simulink model "SF009A_DutyCycThermProtn"  (R2013b)
settings: Solver=FixedStepDiscrete  SolverMode=SingleTasking  StartTime=0.0  StopTime=1  FixedStep=0.1  RelTol=1e-3
values from neighbouring files (symbols this model uses):
  AbsltTThermLimCnt = DataDict.NTC    [SF009A_DutyCycThermProtn_DataDict.m]
  ARCHGLBPRM_100MILLISEC_SEC_F32 = DataDict.Constant    [SF009A_DutyCycThermProtn_DataDict.m]
  CTRLRANDCUTFLT_CNT_U08 = DataDict.Constant    [SF009A_DutyCycThermProtn_DataDict.m]
  CTRLRTFLT_CNT_U08 = DataDict.Constant    [SF009A_DutyCycThermProtn_DataDict.m]
  CUTFLT_CNT_U08 = DataDict.Constant    [SF009A_DutyCycThermProtn_DataDict.m]
  DITHERMLIM_MOTNWTMTR_F32 = DataDict.Constant    [SF009A_DutyCycThermProtn_DataDict.m]
  DutyCycExcddCnt = DataDict.NTC    [SF009A_DutyCycThermProtn_DataDict.m]
  DutyCycThermProtnAbsltCtrlTTblX = DataDict.Calibration    [SF009A_DutyCycThermProtn_DataDict.m]
  DutyCycThermProtnAbsltCtrlTTqTblY = DataDict.Calibration    [SF009A_DutyCycThermProtn_DataDict.m]
  DutyCycThermProtnAbsltCuTTblX = DataDict.Calibration    [SF009A_DutyCycThermProtn_DataDict.m]
  DutyCycThermProtnAbsltCuTTqTblY = DataDict.Calibration    [SF009A_DutyCycThermProtn_DataDict.m]
  DutyCycThermProtnAbsltMotVelBreakPt = DataDict.Calibration    [SF009A_DutyCycThermProtn_DataDict.m]
  DutyCycThermProtnAbsltTTqSlewHiLim = DataDict.Calibration    [SF009A_DutyCycThermProtn_DataDict.m]
  DutyCycThermProtnAbsltTTqSlewLoLim = DataDict.Calibration    [SF009A_DutyCycThermProtn_DataDict.m]
  DutyCycThermProtnCtrlT = DataDict.Calibration    [SF009A_DutyCycThermProtn_DataDict.m]
  DutyCycThermProtnCtrlTSeln = DataDict.Calibration    [SF009A_DutyCycThermProtn_DataDict.m]
  DutyCycThermProtnDutyCycFildThd = DataDict.Calibration    [SF009A_DutyCycThermProtn_DataDict.m]
  DutyCycThermProtnIgnOffCtrlEna = DataDict.Calibration    [SF009A_DutyCycThermProtn_DataDict.m]
  DutyCycThermProtnIgnOffMsgWaitTi = DataDict.Calibration    [SF009A_DutyCycThermProtn_DataDict.m]
  DutyCycThermProtnLstTblValNonStall = DataDict.Calibration    [SF009A_DutyCycThermProtn_DataDict.m]
  DutyCycThermProtnLstTblValStall = DataDict.Calibration    [SF009A_DutyCycThermProtn_DataDict.m]
  DutyCycThermProtnMotPrTSeln = DataDict.Calibration    [SF009A_DutyCycThermProtn_DataDict.m]
  DutyCycThermProtnMplr1NonStallTblY = DataDict.Calibration    [SF009A_DutyCycThermProtn_DataDict.m]
  DutyCycThermProtnMplr1StallTblY = DataDict.Calibration    [SF009A_DutyCycThermProtn_DataDict.m]
  DutyCycThermProtnMplr2NonStallTblY = DataDict.Calibration    [SF009A_DutyCycThermProtn_DataDict.m]
  DutyCycThermProtnMplr2StallTblY = DataDict.Calibration    [SF009A_DutyCycThermProtn_DataDict.m]
  DutyCycThermProtnMplr3NonStallTblY = DataDict.Calibration    [SF009A_DutyCycThermProtn_DataDict.m]
  DutyCycThermProtnMplr3StallTblY = DataDict.Calibration    [SF009A_DutyCycThermProtn_DataDict.m]
  DutyCycThermProtnMplr4NonStallTblY = DataDict.Calibration    [SF009A_DutyCycThermProtn_DataDict.m]
  DutyCycThermProtnMplr4StallTblY = DataDict.Calibration    [SF009A_DutyCycThermProtn_DataDict.m]
  DutyCycThermProtnMplr5NonStallTblY = DataDict.Calibration    [SF009A_DutyCycThermProtn_DataDict.m]
  DutyCycThermProtnMplr5StallTblY = DataDict.Calibration    [SF009A_DutyCycThermProtn_DataDict.m]
  DutyCycThermProtnMplr6NonStallTblY = DataDict.Calibration    [SF009A_DutyCycThermProtn_DataDict.m]
  DutyCycThermProtnMplr6StallTblY = DataDict.Calibration    [SF009A_DutyCycThermProtn_DataDict.m]
  DutyCycThermProtnMplrTblX = DataDict.Calibration    [SF009A_DutyCycThermProtn_DataDict.m]
  DutyCycThermProtnMplrTSeln = DataDict.Calibration    [SF009A_DutyCycThermProtn_DataDict.m]
  DutyCycThermProtnSlowFilTSeln = DataDict.Calibration    [SF009A_DutyCycThermProtn_DataDict.m]
  DutyCycThermProtnThermLimScaFac = DataDict.Calibration    [SF009A_DutyCycThermProtn_DataDict.m]
  DutyCycThermProtnThermLoadLimTblX = DataDict.Calibration    [SF009A_DutyCycThermProtn_DataDict.m]
  DutyCycThermProtnThermLoadLimTblY = DataDict.Calibration    [SF009A_DutyCycThermProtn_DataDict.m]
  DutyCycThermProtnTqCmdSlewDwn = DataDict.Calibration    [SF009A_DutyCycThermProtn_DataDict.m]
  DutyCycThermProtnTqCmdSlewUp = DataDict.Calibration    [SF009A_DutyCycThermProtn_DataDict.m]
  FILVALMIN_ULS_F32 = DataDict.Constant    [SF009A_DutyCycThermProtn_DataDict.m]
  IGNTIOFFTHD_CNT_F32 = DataDict.Constant    [SF009A_DutyCycThermProtn_DataDict.m]
  NODEBSTEP_CNT_U16 = DataDict.Constant    [SF009A_DutyCycThermProtn_DataDict.m]
  ONEPERC_ULS_F32 = DataDict.Constant    [SF009A_DutyCycThermProtn_DataDict.m]
  TAU3_SEC_F32 = DataDict.Constant    [SF009A_DutyCycThermProtn_DataDict.m]
  TAU4_SEC_F32 = DataDict.Constant    [SF009A_DutyCycThermProtn_DataDict.m]
  TAU5_SEC_F32 = DataDict.Constant    [SF009A_DutyCycThermProtn_DataDict.m]
  TAU6_SEC_F32 = DataDict.Constant    [SF009A_DutyCycThermProtn_DataDict.m]
  THERMLOADLIMTBLIDX_ULS_U08 = DataDict.Constant    [SF009A_DutyCycThermProtn_DataDict.m]
undefined symbols (not defined in the file or in its folder): NtcSts1, NvmGetErrSts1
libraries: FixdToFloat x13, Fil x12, NxtrLim x12, simulink x11, NxtrMath x8, FloatToFixd x6, NxtrMax x6, NxtrMin x3, NxtrAbslt x2, NxtrNvM x1
(part 1 of 7)
Description:
  | The purpose of the Thermal Duty Cycle Protection is to limit and protect the system from excessive use,
  | based on motor rotational velocity and system temperature.  It also provides protection status information
  | for use by other functions.
settings Model: ModifiedComment=FZG88Y -- Mon Sep 21 16:56:40 2015 -- Version 1.0.0  Creator=Sneha Pegdal (KPIT)  LastModifiedBy=XZ3VZ1
settings Model: ModifiedHistory=|
  | FZG88Y -- Mon Sep 21 16:56:40 2015 -- Version 1.0.0
  | 
  | 
  | FZG88Y -- Mon Sep 21 16:56:00 2015 -- Version 1.0.0
  | 
  | 
  | FZG88Y -- Mon Sep 21 16:52:01 2015 -- Version 1.0.0
  | 
  | 
  | FZG88Y -- Mon Sep 21 16:48:28 2015 -- Version 1.0.0
  | 
  | 
  | FZG88Y -- Mon Sep 21 16:47:37 2015 -- Version 1.0.0
  | 
  | 
  | FZG88Y -- Mon Sep 21 16:41:44 2015 -- Version 1.0.0
  | 
  | 
  | FZG88Y -- Mon Sep 21 16:36:27 2015 -- Version 1.0.0
  | 
  | 
  | FZG88Y -- Mon Sep 21 16:26:16 2015 -- Version 1.0.0
  | 
  | 
  | FZG88Y -- Mon Sep 21 16:06:23 2015 -- Version 1.0.0
  | 
  | 
  | FZG88Y -- Mon Sep 21 15:59:45 2015 -- Version 1.0.0
  | 
  | 
  | FZG88Y -- Mon Sep 21 15:59:36 2015 -- Version 1.0.0
  | 
  | 
  | FZG88Y -- Mon Sep 21 15:57:42 2015 -- Version 1.0.0
  | 
  | 
  | FZG88Y -- Mon Sep 21 15:57:16 2015 -- Version 1.0.0
  | 
  | 
  | FZG88Y -- Mon Sep 21 15:22:48 2015 -- Version 1.0.0
  | 
  | 
  | FZG88Y -- Mon Sep 21 15:21:30 2015 -- Version 1.0.0
  | 
  | 
  | FZG88Y -- Mon Sep 21 15:21:08 2015 -- Version 1.0.0
  | 
  | 
  | FZG88Y -- Mon Sep 21 15:17:40 2015 -- Version 1.0.0
  | 
  | 
  | FZG88Y -- Mon Sep 21 15:16:45 2015 -- Version 1.0.0
settings SolverCC: AutoInsertRateTranBlk=on  InsertRTBMode=Always
settings DataIOCC: LimitDataPoints=off  SaveFormat=Structure  ReturnWorkspaceOutputs=on
settings OptimizationCC: BlockReduction=off  InlineParams=on  ZeroExternalMemoryAtStartup=off  ZeroInternalMemoryAtStartup=off  OptimizeModelRefInitCode=on  LifeSpan=1
settings DebuggingCC: SignalInfNanChecking=error  SignalRangeChecking=warning  UnderspecifiedInitializationDetection=Simplified  SolverPrmCheckMsg=error  InheritedTsInSrcMsg=error  DiscreteInheritContinuousMsg=error  SingleTaskRateTransMsg=error  TasksWithSamePriorityMsg=error  SigSpecEnsureSampleTimeMsg=error  CheckMatrixSingularityMsg=error  ParameterUnderflowMsg=error  ParameterPrecisionLossMsg=error  ParameterTunabilityLossMsg=error  FixptConstUnderflowMsg=warning  FixptConstOverflowMsg=warning  VectorMatrixConversionMsg=error  SignalLabelMismatchMsg=error  UnconnectedInputMsg=error  UnconnectedOutputMsg=error  UnconnectedLineMsg=error  SFcnCompatibilityMsg=error  UniqueDataStoreMsg=warning  BusObjectLabelMismatch=error  RootOutportRequireBusObject=error  AssertControl=DisableAll  ModelReferenceIOMsg=error  ModelReferenceVersionMismatchMessage=warning  ModelReferenceIOMismatchMessage=error  ModelReferenceCSMismatchMessage=warning  ModelReferenceDataLoggingMessage=error  StateNameClashWarn=warning  StrictBusMsg=ErrorOnBusTreatedAsVector  NonBusSignalsTreatedAsBus=error  SFUnexpectedBacktrackingDiag=error  SFInvalidInputDataAccessInChartInitDiag=error  SFNoUnconditionalDefaultTransitionDiag=error  SFTransitionOutsideNaturalParentDiag=error  SFUnconditionalTransitionShadowingDiag=error  SFUndirectedBroadcastEventsDiag=error
settings ModelReferenceCC: ModelReferenceNumInstancesAllowed=Single
settings RTWCC: SystemTargetFile=autosar.tlc  GenCodeOnly=on  TemplateMakefile=ert_default_tmf  Description=AUTOSAR  GenerateReport=on  ProcessScript=autosar_make_rtw_hook  LaunchReport=on
settings CodeAppCC: GenerateComments=off  IgnoreCustomStorageClasses=off  CustomSymbolStrType=$N$R$M  CustomSymbolStrBlkIO=$N$M  SimulinkBlockComments=off
settings STFCustomTargetCC: ParMdlRefBuildCompliant=on  CompOptLevelCompliant=on  IncludeMdlTerminateFcn=off  CombineOutputUpdateFcns=on  SuppressErrorStatus=on  ERTFirstTimeCompliant=on  ERTCustomFileBanners=on  SupportNonFinite=off  SupportComplex=off  SupportContinuousTime=off  SupportNonInlinedSFcns=off  MATLABClassNameForMDSCustomization=Simulink.SoftwareTarget.ERTCustomization  AutosarCompliant=on  GRTInterface=off  SystemTargetFile=autosar.tlc
settings ERTTargetCC: CodeReplacementLibrary=ANSI_C  ConcurrentExecutionCompliant=off  IncludeMdlTerminateFcn=off  SuppressErrorStatus=on  SupportNonFinite=off  SupportComplex=off  ModelStepFunctionPrototypeControlCompliant=off  CPPClassGenCompliant=off  AutosarCompliant=on  InlinedParameterPlacement=NonHierarchical  ERTCustomFileTemplate=example_file_process.tlc  EnableUserReplacementTypes=on

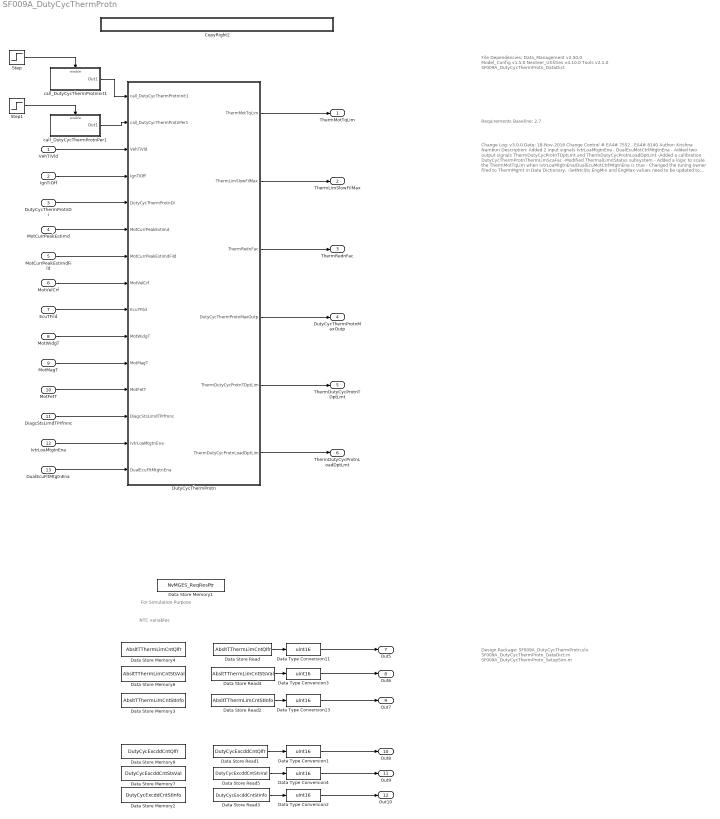
== system SF009A_DutyCycThermProtn ==
  note: For Simulation Purpose
  note: Requirements Baseline: 2.7
  note: File Dependencies:
      |
      | Data_Management v2.50.0
      | Model_Config v1.5.0
      | Nexteer_Utilities v4.10.0
      | Tools v2.1.0
      | SF009A_DutyCycThermProtn_DataDict
  note: Design Package:
      |
      | SF009A_DutyCycThermProtn.slx
      |
      | SF009A_DutyCycThermProtn_DataDict.m
      |
      | SF009A_DutyCycThermProtn_SetupSim.m
  note: NTC variables
  note: Change Log:
      |
      | v3.0.0
      | Date: 18-Nov-2016
      | Change Control # EA4# 7552 , EA4# 8140
      | Author: Krishna Namburi
      | Description:
      | Added 2 input signals IvtrLoaMtgtnEna , DualEcuMotCtrlMtgtnEna
      | - Added two output signals ThermDutyCycProtnTDptLmt and
      | ThermDutyCycProtnLoadDptLmt
      | -Added a calibration DutyCycThermProtnThermLimScaFac
      | -Modified ThermalLimitStatus subsystem
      | - Added a logic to scale the ThermMotTqLim when IvtrLoaMtgtnEna/DualEcuMotCtrlMtgtnEna is true
      | - Changed the tuning owner filed to ThermMgmt in Data Dictionary.
      | -SetNtcSts EngMin and EngMax values need to be updated to match current definition.
      |
      | v2.2.1
      | Date: 21-Sep-2016
      | Change Control # EA4# 7661
      | Author: Krishna Namburi
      | Description:
      | -Added the annotation for look up tables in Multiplier subsystem for
      | Nonstall condition and Stall condition.
      |
      | v2.2.0
      | Date: 05-Aug-2016
      | Change Control #: EA4#6545
      | Author: Fei Yuan
      | Description:
      | - Changed DutyCycThermProtnMplrTblX.Monotony to 'Strictly_Increasing'.
      | - Changed NVM FilStVal.EngInit to blank.
      | - Changed the value of constant CTRLRTFLT_CNT_U08,
      |   CUTFLT_CNT_U08, CTRLRANDCUTFLT_CNT_U08
      | - Added constant NODEBSTEP_CNT_U16
      | - Specified correct bits used in NTCNR_0X0A4 One Pager with new logic to
      |   reach thefull coverage of the MIL test.
      | - Set priority in Init blocks.
      | - Changed NTC names from NTCNR_0X0A3 and NTCNR_0X0A4 to
      |   DutyCycExcddCnt and AbsltTThermLimCnt.
      | - Changed the one-based indexing selectors to zero-based indexing, and
      |   matched the codes.
      | - Changed the DebStep from 0 to NODEBSTEP_CNT_U16 and changed
      |   AbsltTThermLimCnt.NtcTyp to 'None'.
      |
      |
      | v2.1.0
      | Date: 20-Apr-2016
      | Change Control #: EA4#5441
      | Author: Sudeep Shankar
      | Description:
      | - Changed NtcNr1.NTCNR_0X0A4 states:
      | a. 'Prepassed' to 'Passed' and  'Prefailed' to 'Failed' and set debounce step
      | to 0 in the below path:
      | /DutyCycThermProtn/DutyCycThermProtnPer1/TempratureLimiting
      |
      | - Removed ABSLTTTHERMLIMDIAGPASSSTEP_CNT_U16 and
      | ABSLTTTHERMLIMDIAGFAILSTEP_CNT_U16 from DataDictionary as
      | these constants are no longer used.
      |
      | - In Init block, GetErrorStatus block library block is used instead of
      | hardcoded '0' setting to verify NVM validity.
      |
      | - Requirement links to SF009A_132,133,178,179,140 removed as they
      | are no longer applicable
      | - Created requirement links to SF009A_285 and SF009A_138.
      |
      | v2.0.0
      | Date: 04-Apr-2016
      | Change Control #: EA4#5077, EA4#5088
      | Author: Sudeep Shankar
      | Description:
      | EA4#5088:
      | - Removed the calibration DutyCycThermProtnDftIgnOffTi and set
      | the state variables to FILVALMIN_ULS_F32 (0) in the below path:
      | /DutyCycThermProtnPer1/ServiceDefeatFiltSVReinit
      | - Removed DutyCycThermProtnDftIgnOffTi from the DataDictionary.
      |
      | - Constant '0' is changed to defined constant "FILVALMIN_ULS_F32" in
      | the path given below:
      | a.  /DutyCycThermProtnInit1/PowerOnTasks/DefaultIgnOffTime
      | b.  /DutyCycThermProtnPer1/FiltSVReinit/VehTiVldDisabled
      |
      | EA4#5077:
      | -DutyCycThermProtnMaxOutp is added as an output and DataDictionary
      | is updated to include the output signal definition.
      | - Removed display output dDutyCycThermProtnMaxOutp from
      | design and DataDictionary
      |
      | v1.3.0
      | Date: 01-Feb-2015
      | Change Control #: EA4#3601
      | Author: Fei Yuan
      | Description:
      | - Change the logic of NTCs and modify the NTCs definition in the Data
      |   Dictionary.
      | - Add constants CTRLRANDCUTFLT_CNT_U08, CTRLRTFLT_CNT_U08,
      |   CUTFLT_CNT_U08 for NTC.
      |
      | v 1.2.0
      | Date: 09-Dec-2015
      | Chang Control #: EA4#2444
      | Author: Fei Yuan
      | Description
      | - Fixing the the anomaly caused by a floating point exception error by
      |   redesign the logic in PowerOnTasks function and FiltSVReint function.
      | - One constant IGNTIOFFTHD_CNT_F32 is added.
      |
      | v1.1.0
      | Date: 08-Oct-2015
      | Change Control #: EA4#656 (Task EA4#4118)
      | DRW:  Sneha Pegdal/Muragesh Asundi (KPIT)
      | Description:
      | - Data type conversion from float32 to fixed and fixed to float32 before
      |   and after interpolation tables
      | - Debounce logic implemented for NTC 0X0A4
      | - Range limiter added for output ThermRednFac
      | - PIM 'LstTblValRateLimrStVari' is initialized in init function
      |
      | v1.0.0
      | Date: 21-Sept-2015
      | Change Control #: EA4#656 (Task EA4#3734)
      | DRW:  Sneha Pegdal/Muragesh Asundi
      | Description:
      | - Initial Release of EA4 1.0.0 from EA3 V014
  VehTiVld : Inport
  IgnTiOff : Inport  Port=2
  DutyCycThermProtnDi : Inport  Port=3
  MotCurrPeakEstimd : Inport  Port=4
  MotCurrPeakEstimdFild : Inport  Port=5
  MotVelCrf : Inport  Port=6
  EcuTFild : Inport  Port=7
  MotWidgT : Inport  Port=8
  MotMagT : Inport  Port=9
  MotFetT : Inport  Port=10
  DiagcStsLimdTPrfmnc : Inport  Port=11
  IvtrLoaMtgtnEna : Inport  Port=12
  DualEcuFltMtgtnEna : Inport  Port=13
  CopyRight2 : Subsystem  Description=|  mask(Copyright Information){none=on}
      | Copyright info block.                                               
      |                                                                     
      | Place copyright information at the top of every subsystem in design.
      mask prompts: none "No parameters"
      mask help: Place copyright information at the top of every subsystem in design.
      mask Display:
      | NxtrConf = 'Nexteer Confidential';
      | 
      | sys = bdroot; %handle for the current model ("system")
      | first = get_param(sys,'Created');
      | first = first(end-3:end);  %year is last four digits
      | 
      | last = get_param(sys,'LastModifiedDate');
      | if isempty(last)
      |     last = datestr(now,'yyyy');
      | else
      |     last = last(end-3:end);
      | end
      | 
      | if strcmp(first,last)
      |     fprintf('%s -- Copyright %s Nexteer',NxtrConf,first)
      | else
      |     fprintf('%s -- %s%s- %s Nexteer',NxtrConf,char(169),first,last)
      | end
  Data Store Memory1 : DataStoreMemory  DataStoreName=NvMGES_ReqResPtr  OutDataTypeStr=uint8
  Data Store Read : DataStoreRead  DataStoreName=AbsltTThermLimCntQlfr  SampleTime=0.1
  Data Store Read1 : DataStoreRead  DataStoreName=DutyCycExcddCntQlfr  SampleTime=0.1
  Data Store Read2 : DataStoreRead  DataStoreName=AbsltTThermLimCntStInfo  SampleTime=0.1
  Data Store Read3 : DataStoreRead  DataStoreName=DutyCycExcddCntStInfo  SampleTime=0.1
  Data Store Read4 : DataStoreRead  DataStoreName=AbsltTThermLimCntStsVal  SampleTime=0.1
  Data Store Read5 : DataStoreRead  DataStoreName=DutyCycExcddCntStsVal  SampleTime=0.1
  Data Store Memory2 : DataStoreMemory  DataStoreName=DutyCycExcddCntStInfo
  Data Store Memory3 : DataStoreMemory  DataStoreName=AbsltTThermLimCntStInfo
  Data Store Memory4 : DataStoreMemory  DataStoreName=AbsltTThermLimCntQlfr  InitialValue=SigQlfr1.SIGQLFR_NORES  OutDataTypeStr=Enum: SigQlfr1
  Data Store Memory6 : DataStoreMemory  DataStoreName=AbsltTThermLimCntStsVal  InitialValue=NtcSts1.NTCSTS_PASSD  OutDataTypeStr=Enum: NtcSts1
  Data Store Memory7 : DataStoreMemory  DataStoreName=DutyCycExcddCntStsVal  InitialValue=NtcSts1.NTCSTS_PASSD  OutDataTypeStr=Enum: NtcSts1
  Data Store Memory9 : DataStoreMemory  DataStoreName=DutyCycExcddCntQlfr  InitialValue=SigQlfr1.SIGQLFR_NORES  OutDataTypeStr=Enum: SigQlfr1
  Data Type Conversion{1..4,11,13} (6 alike) : DataTypeConversion  OutDataTypeStr=uint16
  DutyCycThermProtn : Subsystem
  Step : Step  Before=1  After=0  SampleTime=0.1
  Step1 : Step  SampleTime=0.1
  call_DutyCycThermProtnInit1 : Subsystem  TreatAsAtomicUnit=on
  call_DutyCycThermProtnPer1 : Subsystem  TreatAsAtomicUnit=on
  ThermMotTqLim : Outport
  ThermLimSlowFilMax : Outport  Port=2
  ThermRednFac : Outport  Port=3
  DutyCycThermProtnMaxOutp : Outport  Port=4
  ThermDutyCycProtnTDptLmt : Outport  Port=5
  ThermDutyCycProtnLoadDptLmt : Outport  Port=6
  Out5 : Outport  Port=7
  Out6 : Outport  Port=8
  Out7 : Outport  Port=9
  Out8 : Outport  Port=10
  Out9 : Outport  Port=11
  Out10 : Outport  Port=12
  wires:
  DutyCycThermProtn/1(ThermMotTqLim) -> ThermMotTqLim/1
  DutyCycThermProtn/2(ThermLimSlowFilMax) -> ThermLimSlowFilMax/1
  DutyCycThermProtn/3(ThermRednFac) -> ThermRednFac/1
  VehTiVld/1 -> DutyCycThermProtn/3(VehTiVld)
  IgnTiOff/1 -> DutyCycThermProtn/4(IgnTiOff)
  DutyCycThermProtnDi/1 -> DutyCycThermProtn/5(DutyCycThermProtnDi)
  MotCurrPeakEstimd/1 -> DutyCycThermProtn/6(MotCurrPeakEstimd)
  MotCurrPeakEstimdFild/1 -> DutyCycThermProtn/7(MotCurrPeakEstimdFild)
  MotVelCrf/1 -> DutyCycThermProtn/8(MotVelCrf)
  EcuTFild/1 -> DutyCycThermProtn/9(EcuTFild)
  MotWidgT/1 -> DutyCycThermProtn/10(MotWidgT)
  MotMagT/1 -> DutyCycThermProtn/11(MotMagT)
  MotFetT/1 -> DutyCycThermProtn/12(MotFetT)
  DiagcStsLimdTPrfmnc/1 -> DutyCycThermProtn/13(DiagcStsLimdTPrfmnc)
  Data Store Read/1 -> Data Type Conversion11/1
  Data Store Read2/1 -> Data Type Conversion13/1
  Data Type Conversion13/1 -> Out7/1
  Data Type Conversion11/1 -> Out5/1
  Data Store Read1/1 -> Data Type Conversion1/1
  Data Store Read3/1 -> Data Type Conversion2/1
  Data Type Conversion2/1 -> Out10/1
  Data Type Conversion1/1 -> Out8/1
  Data Store Read4/1 -> Data Type Conversion3/1
  Data Type Conversion3/1 -> Out6/1
  Data Store Read5/1 -> Data Type Conversion4/1
  Data Type Conversion4/1 -> Out9/1
  DutyCycThermProtn/4(DutyCycThermProtnMaxOutp) -> DutyCycThermProtnMaxOutp/1
  Step/1 -> call_DutyCycThermProtnInit1/Enable
  Step1/1 -> call_DutyCycThermProtnPer1/Enable
  call_DutyCycThermProtnInit1/1(Out1) -> DutyCycThermProtn/1(call_DutyCycThermProtnInit1)
  call_DutyCycThermProtnPer1/1(Out1) -> DutyCycThermProtn/2(call_DutyCycThermProtnPer1)
  DutyCycThermProtn/5(ThermDutyCycProtnTDptLim) -> ThermDutyCycProtnTDptLmt/1
  DutyCycThermProtn/6(ThermDutyCycProtnLoadDptLim) -> ThermDutyCycProtnLoadDptLmt/1
  IvtrLoaMtgtnEna/1 -> DutyCycThermProtn/14(IvtrLoaMtgtnEna)
  DualEcuFltMtgtnEna/1 -> DutyCycThermProtn/15(DualEcuFltMtgtnEna)

== system SF009A_DutyCycThermProtn/CopyRight2 ==

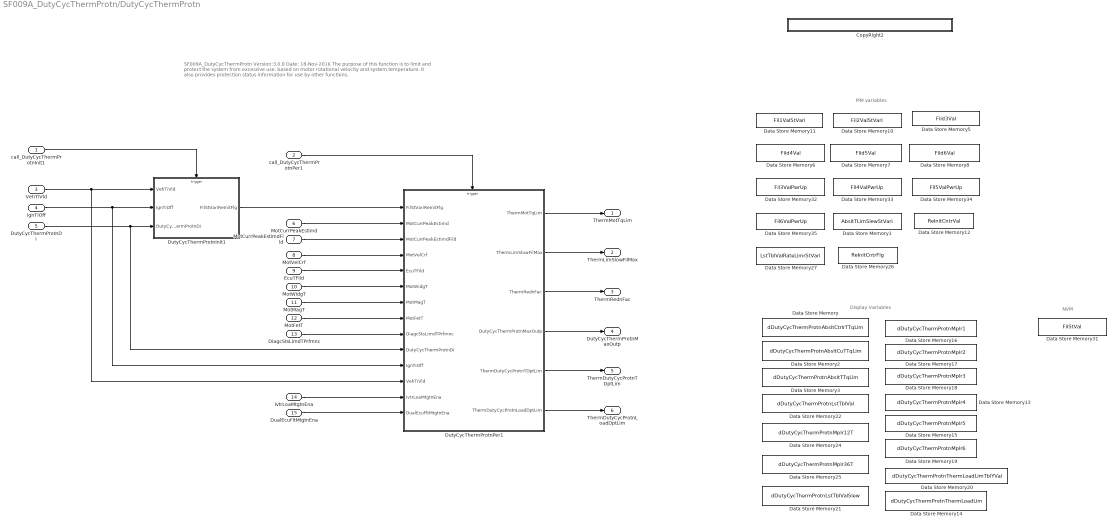
== system SF009A_DutyCycThermProtn/DutyCycThermProtn ==
  note: NVM
  note: Display Variables
  note: PIM variables
  note: SF009A_DutyCycThermProtn      Version:3.0.0                                                 Date:  18-Nov-2016
      | The purpose of this function is to limit and protect the system from excessive use, based on motor rotational velocity and system temperature.
      | It also provides protection status information for use by other functions.
  call_DutyCycThermProtnInit1 : Inport
  call_DutyCycThermProtnPer1 : Inport  Port=2
  VehTiVld : Inport  RequirementInfo={'linktype_rmi_doors' '0000a52a (/E-STEER Core/SubSystem Specifications/Application Functions/SF009A Thermal Duty Cycle Protection)' '#SF009A_39' 'true' 'REQ: SF009A_39' '' } %GIDa_864c1118_778d_4343_bc4d_3cc30f47fe32  Port=3
  IgnTiOff : Inport  RequirementInfo={'linktype_rmi_doors' '0000a52a (/E-STEER Core/SubSystem Specifications/Application Functions/SF009A Thermal Duty Cycle Protection)' '#SF009A_38' 'true' 'REQ: SF009A_38' '' } %GIDa_91c1f96a_b6bf_4566_a475_97c670e9d476  Port=4
  DutyCycThermProtnDi : Inport  RequirementInfo={'linktype_rmi_doors' '0000a52a (/E-STEER Core/SubSystem Specifications/Application Functions/SF009A Thermal Duty Cycle Protection)' '#SF009A_41' 'true' 'REQ: SF009A_41' '' } %GIDa_52de0261_92a3_4db5_85ad_f2cfdd3afac9  Port=5
  MotCurrPeakEstimd : Inport  RequirementInfo={'linktype_rmi_doors' '0000a52a (/E-STEER Core/SubSystem Specifications/Application Functions/SF009A Thermal Duty Cycle Protection)' '#SF009A_9' 'true' 'REQ: SF009A_9' '' } %GIDa_eb01aa28_247f_476b_b7cf_89c03dfe9b33  Port=6
  MotCurrPeakEstimdFild : Inport  RequirementInfo={'linktype_rmi_doors' '0000a52a (/E-STEER Core/SubSystem Specifications/Application Functions/SF009A Thermal Duty Cycle Protection)' '#SF009A_32' 'true' 'REQ: SF009A_32' '' } %GIDa_9a670469_cfaf_4df7_a178_0c897feeb23b  Port=7
  MotVelCrf : Inport  RequirementInfo={'linktype_rmi_doors' '0000a52a (/E-STEER Core/SubSystem Specifications/Application Functions/SF009A Thermal Duty Cycle Protection)' '#SF009A_33' 'true' 'REQ: SF009A_33' '' } %GIDa_17006e69_4cbc_4e82_acf3_d666e95c1429  Port=8
  EcuTFild : Inport  RequirementInfo={'linktype_rmi_doors' '0000a52a (/E-STEER Core/SubSystem Specifications/Application Functions/SF009A Thermal Duty Cycle Protection)' '#SF009A_34' 'true' 'REQ: SF009A_34' '' } %GIDa_c8c2b021_b73b_4c92_8ccd_6e5a076a1f2a  Port=9
  MotWidgT : Inport  RequirementInfo={'linktype_rmi_doors' '0000a52a (/E-STEER Core/SubSystem Specifications/Application Functions/SF009A Thermal Duty Cycle Protection)' '#SF009A_37' 'true' 'REQ: SF009A_37' '' } %GIDa_9410e4a6_6429_4607_8605_4053cc1d35e0  Port=10
  MotMagT : Inport  RequirementInfo={'linktype_rmi_doors' '0000a52a (/E-STEER Core/SubSystem Specifications/Application Functions/SF009A Thermal Duty Cycle Protection)' '#SF009A_36' 'true' 'REQ: SF009A_36' '' } %GIDa_fbe04a47_e117_41dd_aa1c_e1d39b0f3863  Port=11
  MotFetT : Inport  RequirementInfo={'linktype_rmi_doors' '0000a52a (/E-STEER Core/SubSystem Specifications/Application Functions/SF009A Thermal Duty Cycle Protection)' '#SF009A_35' 'true' 'REQ: SF009A_35' '' } %GIDa_71f8b7c1_ac64_4dbe_9e4e_6077f5ec5b92  Port=12
  DiagcStsLimdTPrfmnc : Inport  RequirementInfo={} %GIDa_5be0298f_407d_4486_aa28_f0641ea2ee13  Port=13
  IvtrLoaMtgtnEna : Inport  RequirementInfo={} %GIDa_95a98e68_beb4_4b72_8a6c_64a623d70b4b  Port=14
  DualEcuFltMtgtnEna : Inport  RequirementInfo={} %GIDa_064281bc_c4a7_4daa_abcd_ffd5837e9fb5  Port=15
  CopyRight2 : Subsystem  Description=|  mask(Copyright Information){none=on}
      | Copyright info block.                                               
      |                                                                     
      | Place copyright information at the top of every subsystem in design.
      mask prompts: none "No parameters"
      mask help: Place copyright information at the top of every subsystem in design.
      mask Display:
      | NxtrConf = 'Nexteer Confidential';
      | 
      | sys = bdroot; %handle for the current model ("system")
      | first = get_param(sys,'Created');
      | if(isempty(first))
      |     first = datestr(now,'yyyy');
      | else
      |     first = first(end-3:end);  %year is last four digits
      | end
      | 
      | last = get_param(sys,'LastModifiedDate');
      | if isempty(last)
      |     last = datestr(now,'yyyy');
      | else
      |     last = last(end-3:end);
      | end
      | 
      | if strcmp(first,last)
      |     fprintf('%s -- Copyright %s Nexteer',NxtrConf,first)
      | else
      |     fprintf('%s -- %s%s- %s Nexteer',NxtrConf,char(169),first,last)
      | end
  Data Store Memory : DataStoreMemory  DataStoreName=dDutyCycThermProtnAbsltCtrlrTTqLim  ReadBeforeWriteMsg=warning  WriteAfterWriteMsg=warning  WriteAfterReadMsg=warning  StateMustResolveToSignalObject=on
  Data Store Memory1 : DataStoreMemory  DataStoreName=AbsltTLimSlewStVari  StateMustResolveToSignalObject=on
      settings: AttributesFormatString=Initial Value: %<InitialValue>
  Data Store Memory10 : DataStoreMemory  DataStoreName=Fil2ValStVari  InitialValue=[]  StateMustResolveToSignalObject=on
      settings: AttributesFormatString=Initial Value: %<InitialValue>
  Data Store Memory11 : DataStoreMemory  DataStoreName=Fil1ValStVari  InitialValue=[]  StateMustResolveToSignalObject=on
      settings: AttributesFormatString=Initial Value: %<InitialValue>
  Data Store Memory12 : DataStoreMemory  DataStoreName=ReInitCntrVal  InitialValue=[]  StateMustResolveToSignalObject=on
  Data Store Memory13 : DataStoreMemory  DataStoreName=dDutyCycThermProtnMplr4  ReadBeforeWriteMsg=warning  WriteAfterWriteMsg=warning  WriteAfterReadMsg=warning  StateMustResolveToSignalObject=on
  Data Store Memory14 : DataStoreMemory  DataStoreName=dDutyCycThermProtnThermLoadLim  ReadBeforeWriteMsg=warning  WriteAfterWriteMsg=warning  WriteAfterReadMsg=warning  StateMustResolveToSignalObject=on
  Data Store Memory15 : DataStoreMemory  DataStoreName=dDutyCycThermProtnMplr5  ReadBeforeWriteMsg=warning  WriteAfterWriteMsg=warning  WriteAfterReadMsg=warning  StateMustResolveToSignalObject=on
  Data Store Memory16 : DataStoreMemory  DataStoreName=dDutyCycThermProtnMplr1  ReadBeforeWriteMsg=warning  WriteAfterWriteMsg=warning  WriteAfterReadMsg=warning  StateMustResolveToSignalObject=on
  Data Store Memory17 : DataStoreMemory  DataStoreName=dDutyCycThermProtnMplr2  ReadBeforeWriteMsg=warning  WriteAfterWriteMsg=warning  WriteAfterReadMsg=warning  StateMustResolveToSignalObject=on
  Data Store Memory18 : DataStoreMemory  DataStoreName=dDutyCycThermProtnMplr3  ReadBeforeWriteMsg=warning  WriteAfterWriteMsg=warning  WriteAfterReadMsg=warning  StateMustResolveToSignalObject=on
  Data Store Memory19 : DataStoreMemory  DataStoreName=dDutyCycThermProtnMplr6  ReadBeforeWriteMsg=warning  WriteAfterWriteMsg=warning  WriteAfterReadMsg=warning  StateMustResolveToSignalObject=on
  Data Store Memory2 : DataStoreMemory  DataStoreName=dDutyCycThermProtnAbsltCuTTqLim  ReadBeforeWriteMsg=warning  WriteAfterWriteMsg=warning  WriteAfterReadMsg=warning  StateMustResolveToSignalObject=on
  Data Store Memory20 : DataStoreMemory  DataStoreName=dDutyCycThermProtnThermLoadLimTblYVal  ReadBeforeWriteMsg=warning  WriteAfterWriteMsg=warning  WriteAfterReadMsg=warning  StateMustResolveToSignalObject=on
  Data Store Memory21 : DataStoreMemory  DataStoreName=dDutyCycThermProtnLstTblValSlew  ReadBeforeWriteMsg=warning  WriteAfterWriteMsg=warning  WriteAfterReadMsg=warning  StateMustResolveToSignalObject=on
  Data Store Memory22 : DataStoreMemory  DataStoreName=dDutyCycThermProtnLstTblVal  ReadBeforeWriteMsg=warning  WriteAfterWriteMsg=warning  WriteAfterReadMsg=warning  StateMustResolveToSignalObject=on
  Data Store Memory24 : DataStoreMemory  DataStoreName=dDutyCycThermProtnMplr12T  ReadBeforeWriteMsg=warning  WriteAfterWriteMsg=warning  WriteAfterReadMsg=warning  StateMustResolveToSignalObject=on
  Data Store Memory25 : DataStoreMemory  DataStoreName=dDutyCycThermProtnMplr36T  ReadBeforeWriteMsg=warning  WriteAfterWriteMsg=warning  WriteAfterReadMsg=warning  StateMustResolveToSignalObject=on
  Data Store Memory26 : DataStoreMemory  DataStoreName=ReInitCntrFlg  InitialValue=[]  StateMustResolveToSignalObject=on
  Data Store Memory27 : DataStoreMemory  DataStoreName=LstTblValRateLimrStVari  StateMustResolveToSignalObject=on
      settings: AttributesFormatString=Initial Value: %<InitialValue>
  Data Store Memory3 : DataStoreMemory  DataStoreName=dDutyCycThermProtnAbsltTTqLim  ReadBeforeWriteMsg=warning  WriteAfterWriteMsg=warning  WriteAfterReadMsg=warning  StateMustResolveToSignalObject=on
  Data Store Memory31 : DataStoreMemory  DataStoreName=FilStVal  InitialValue=[]  StateMustResolveToSignalObject=on
      settings: AttributesFormatString=Initial Value: %<InitialValue>
  Data Store Memory32 : DataStoreMemory  DataStoreName=Fil3ValPwrUp  StateMustResolveToSignalObject=on
      settings: AttributesFormatString=Initial Value: %<InitialValue>
  Data Store Memory33 : DataStoreMemory  DataStoreName=Fil4ValPwrUp  StateMustResolveToSignalObject=on
      settings: AttributesFormatString=Initial Value: %<InitialValue>
  Data Store Memory34 : DataStoreMemory  DataStoreName=Fil5ValPwrUp  StateMustResolveToSignalObject=on
      settings: AttributesFormatString=Initial Value: %<InitialValue>
  Data Store Memory35 : DataStoreMemory  DataStoreName=Fil6ValPwrUp  StateMustResolveToSignalObject=on
      settings: AttributesFormatString=Initial Value: %<InitialValue>
  Data Store Memory5 : DataStoreMemory  RequirementInfo={'linktype_rmi_doors' '0000a52a (/E-STEER Core/SubSystem Specifications/Application Functions/SF009A Thermal Duty Cycle Protection)' '#SF009A_285' 'true' 'REQ: SF009A_285' '' } %GIDa_75ef786b_1159_4210_af92_457fb74ea7ff  DataStoreName=Fild3Val  InitialValue=[]  StateMustResolveToSignalObject=on
      settings: AttributesFormatString=Initial Value: %<InitialValue>
  Data Store Memory6 : DataStoreMemory  RequirementInfo={'linktype_rmi_doors' '0000a52a (/E-STEER Core/SubSystem Specifications/Application Functions/SF009A Thermal Duty Cycle Protection)' '#SF009A_285' 'true' 'REQ: SF009A_285' '' } %GIDa_b620ecc7_db63_446e_8f03_37af3e2285f3  DataStoreName=Fild4Val  InitialValue=[]  StateMustResolveToSignalObject=on
      settings: AttributesFormatString=Initial Value: %<InitialValue>
  Data Store Memory7 : DataStoreMemory  RequirementInfo={'linktype_rmi_doors' '0000a52a (/E-STEER Core/SubSystem Specifications/Application Functions/SF009A Thermal Duty Cycle Protection)' '#SF009A_285' 'true' 'REQ: SF009A_285' '' } %GIDa_967c7843_d0f8_4563_990c_866e0e761b03  DataStoreName=Fild5Val  InitialValue=[]  StateMustResolveToSignalObject=on
      settings: AttributesFormatString=Initial Value: %<InitialValue>
  Data Store Memory8 : DataStoreMemory  RequirementInfo={'linktype_rmi_doors' '0000a52a (/E-STEER Core/SubSystem Specifications/Application Functions/SF009A Thermal Duty Cycle Protection)' '#SF009A_285' 'true' 'REQ: SF009A_285' '' } %GIDa_dc28bb5e_67e6_4f32_a254_c55d8b607b43  DataStoreName=Fild6Val  InitialValue=[]  StateMustResolveToSignalObject=on
      settings: AttributesFormatString=Initial Value: %<InitialValue>
  DutyCycThermProtnInit1 : Subsystem  TreatAsAtomicUnit=on
  DutyCycThermProtnPer1 : Subsystem  ClipboardFcn=Priority=%<Priority>  TreatAsAtomicUnit=on
  ThermMotTqLim : Outport  RequirementInfo={'linktype_rmi_doors' '0000a52a (/E-STEER Core/SubSystem Specifications/Application Functions/SF009A Thermal Duty Cycle Protection)' '#SF009A_11' 'true' 'REQ: SF009A_11' '' } %GIDa_b003c252_92e7_4128_b79e_51af7283823f
  ThermLimSlowFilMax : Outport  RequirementInfo={'linktype_rmi_doors' '0000a52a (/E-STEER Core/SubSystem Specifications/Application Functions/SF009A Thermal Duty Cycle Protection)' '#SF009A_44' 'true' 'REQ: SF009A_44' '' } %GIDa_6720560f_cd3f_4a66_9337_c9fda3d2b968  Port=2
  ThermRednFac : Outport  RequirementInfo={'linktype_rmi_doors' '0000a52a (/E-STEER Core/SubSystem Specifications/Application Functions/SF009A Thermal Duty Cycle Protection)' '#SF009A_45' 'true' 'REQ: SF009A_45' '' } %GIDa_bdcba9de_b25d_49eb_95b7_6430acdc662c  Port=3
  DutyCycThermProtnMaxOutp : Outport  RequirementInfo={'linktype_rmi_doors' '0000a52a (/E-STEER Core/SubSystem Specifications/Application Functions/SF009A Thermal Duty Cycle Protection)' '#SF009A_283' 'true' 'REQ: SF009A_283' '' } %GIDa_49eea21d_06a7_40bd_b604_6809298a62bb  Port=4
  ThermDutyCycProtnTDptLim : Outport  RequirementInfo={'linktype_rmi_doors' '0000a52a (/E-STEER Core/SubSystem Specifications/Application Functions/SF009A Thermal Duty Cycle Protection)' '#SF009A_293' 'true' 'REQ: SF009A_293' '' } %GIDa_ce06e884_6156_4583_958e_0184ba4e1972  Port=5
  ThermDutyCycProtnLoadDptLim : Outport  RequirementInfo={'linktype_rmi_doors' '0000a52a (/E-STEER Core/SubSystem Specifications/Application Functions/SF009A Thermal Duty Cycle Protection)' '#SF009A_294' 'true' 'REQ: SF009A_294' '' } %GIDa_34ea47fc_4302_4f6d_8bb6_be5416b6175c  Port=6
  wires:
  call_DutyCycThermProtnPer1/1 -> DutyCycThermProtnPer1/Trigger
  call_DutyCycThermProtnInit1/1 -> DutyCycThermProtnInit1/Trigger
  MotCurrPeakEstimd/1 -> DutyCycThermProtnPer1/2(MotCurrPeakEstimd)
  MotCurrPeakEstimdFild/1 -> DutyCycThermProtnPer1/3(MotCurrPeakEstimdFild)
  MotVelCrf/1 -> DutyCycThermProtnPer1/4(MotVelCrf)
  EcuTFild/1 -> DutyCycThermProtnPer1/5(EcuTFild)
  MotMagT/1 -> DutyCycThermProtnPer1/7(MotMagT)
  DiagcStsLimdTPrfmnc/1 -> DutyCycThermProtnPer1/9(DiagcStsLimdTPrfmnc)
  MotWidgT/1 -> DutyCycThermProtnPer1/6(MotWidgT)
  MotFetT/1 -> DutyCycThermProtnPer1/8(MotFetT)
  VehTiVld/1 -> DutyCycThermProtnInit1/1(VehTiVld), DutyCycThermProtnPer1/12(VehTiVld)
  DutyCycThermProtnPer1/1(ThermMotTqLim) -> ThermMotTqLim/1
  DutyCycThermProtnPer1/2(ThermLimSlowFilMax) -> ThermLimSlowFilMax/1
  DutyCycThermProtnPer1/3(ThermRednFac) -> ThermRednFac/1
  IgnTiOff/1 -> DutyCycThermProtnInit1/2(IgnTiOff), DutyCycThermProtnPer1/11(IgnTiOff)
  DutyCycThermProtnDi/1 -> DutyCycThermProtnPer1/10(DutyCycThermProtnDi), DutyCycThermProtnInit1/3(DutyCycThermProtnDi)
  DutyCycThermProtnInit1/1(FilStVariReInitFlg) -> DutyCycThermProtnPer1/1(FilStVariReInitFlg)
  DutyCycThermProtnPer1/4(DutyCycThermProtnMaxOutp) -> DutyCycThermProtnMaxOutp/1
  DutyCycThermProtnPer1/6(ThermDutyCycProtnLoadDptLim) -> ThermDutyCycProtnLoadDptLim/1
  DutyCycThermProtnPer1/5(ThermDutyCycProtnTDptLim) -> ThermDutyCycProtnTDptLim/1
  IvtrLoaMtgtnEna/1 -> DutyCycThermProtnPer1/13(IvtrLoaMtgtnEna)
  DualEcuFltMtgtnEna/1 -> DutyCycThermProtnPer1/14(DualEcuFltMtgtnEna)

== system SF009A_DutyCycThermProtn/call_DutyCycThermProtnInit1 ==
  Enable : EnablePort
  call_DutyCycThermProtnPer1 : simulink/Ports & Subsystems/Function-Call Generator  RequirementInfo={'linktype_rmi_doors' '0000a52a (/E-STEER Core/SubSystem Specifications/Application Functions/SF009A Thermal Duty Cycle Protection)' '#SF009A_177' 'true' 'REQ: SF009A_177' '' } %GIDa_46b53a92_bc2f_4bf5_be4d_f17ac0a4975c  sample_time=0.1  numberOfIterations=1
  Out1 : Outport
  wires:
  call_DutyCycThermProtnPer1/1 -> Out1/1

== system SF009A_DutyCycThermProtn/call_DutyCycThermProtnPer1 ==
  Enable : EnablePort
  call_DutyCycThermProtnPer1 : simulink/Ports & Subsystems/Function-Call Generator  RequirementInfo={'linktype_rmi_doors' '0000a52a (/E-STEER Core/SubSystem Specifications/Application Functions/SF009A Thermal Duty Cycle Protection)' '#SF009A_177' 'true' 'REQ: SF009A_177' '' } %GIDa_f613af9b_79c2_4a3a_a4a6_2328d4765ebc  sample_time=0.1  numberOfIterations=1
  Out1 : Outport
  wires:
  call_DutyCycThermProtnPer1/1 -> Out1/1

== system SF009A_DutyCycThermProtn/DutyCycThermProtn/CopyRight2 ==

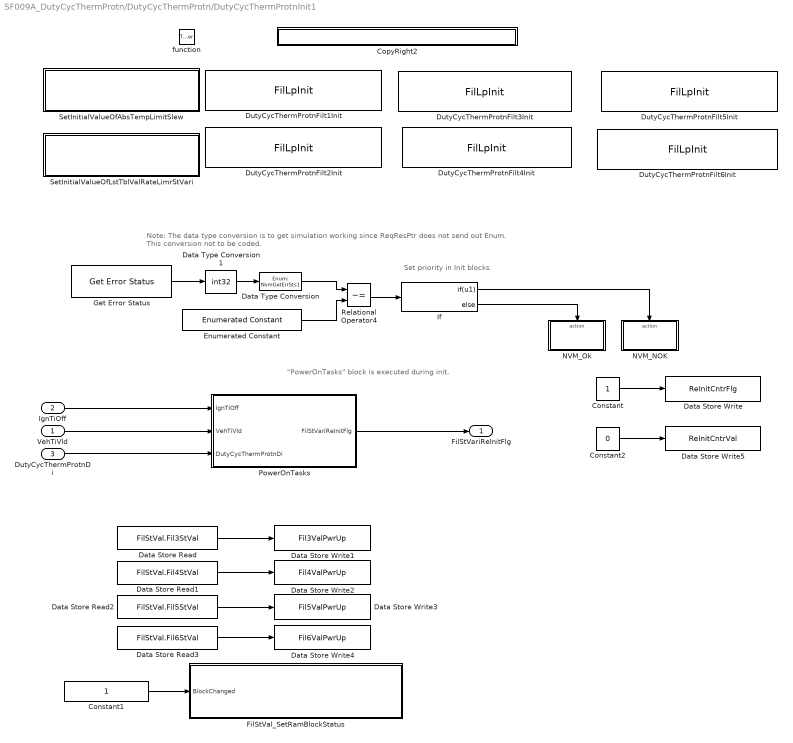
== system SF009A_DutyCycThermProtn/DutyCycThermProtn/DutyCycThermProtnInit1 ==
  note: Set priority in Init blocks
  note: "PowerOnTasks" block is executed during init.
  note: Note: The data type conversion is to get simulation working since ReqResPtr does not send out Enum. This
      | conversion not to be coded.
  VehTiVld : Inport
  IgnTiOff : Inport  Port=2
  DutyCycThermProtnDi : Inport  RequirementInfo={} %GIDa_c6085bca_aa6d_458d_ae20_3753cf3ed8a0  Port=3
  function : TriggerPort  TriggerType=function-call
  Constant : Constant  OutDataTypeStr=Inherit: Inherit via back propagation
  Constant1 : Constant  OutDataTypeStr=boolean
  Constant2 : Constant  Value=0  OutDataTypeStr=Inherit: Inherit via back propagation
  CopyRight2 : Subsystem  Description=|  mask(Copyright Information){none=on}
      | Copyright info block.                                               
      |                                                                     
      | Place copyright information at the top of every subsystem in design.
      mask prompts: none "No parameters"
      mask help: Place copyright information at the top of every subsystem in design.
      mask Display:
      | NxtrConf = 'Nexteer Confidential';
      | 
      | sys = bdroot; %handle for the current model ("system")
      | first = get_param(sys,'Created');
      | first = first(end-3:end);  %year is last four digits
      | 
      | last = get_param(sys,'LastModifiedDate');
      | if isempty(last)
      |     last = datestr(now,'yyyy');
      | else
      |     last = last(end-3:end);
      | end
      | 
      | if strcmp(first,last)
      |     fprintf('%s -- Copyright %s Nexteer',NxtrConf,first)
      | else
      |     fprintf('%s -- %s%s- %s Nexteer',NxtrConf,char(169),first,last)
      | end
  Data Store Read : DataStoreRead  DataStoreName=FilStVal  DataStoreElements=FilStVal.Fil3StVal
  Data Store Read1 : DataStoreRead  DataStoreName=FilStVal  DataStoreElements=FilStVal.Fil4StVal
  Data Store Read2 : DataStoreRead  DataStoreName=FilStVal  DataStoreElements=FilStVal.Fil5StVal
  Data Store Read3 : DataStoreRead  DataStoreName=FilStVal  DataStoreElements=FilStVal.Fil6StVal
  Data Store Write : DataStoreWrite  DataStoreName=ReInitCntrFlg
  Data Store Write1 : DataStoreWrite  DataStoreName=Fil3ValPwrUp
  Data Store Write2 : DataStoreWrite  DataStoreName=Fil4ValPwrUp
  Data Store Write3 : DataStoreWrite  DataStoreName=Fil5ValPwrUp
  Data Store Write4 : DataStoreWrite  DataStoreName=Fil6ValPwrUp
  Data Store Write5 : DataStoreWrite  DataStoreName=ReInitCntrVal
  Data Type Conversion : DataTypeConversion  RequirementInfo={'linktype_rmi_doors' '0000a52a (/E-STEER Core/SubSystem Specifications/Application Functions/SF009A Thermal Duty Cycle Protection)' '#SF009A_285' 'true' 'REQ: SF009A_285' '' } %GIDa_33095d22_a786_4779_9c18_b6ff17e94fe6  OutDataTypeStr=Enum: NvmGetErrSts1
  Data Type Conversion1 : DataTypeConversion  RequirementInfo={'linktype_rmi_doors' '0000a52a (/E-STEER Core/SubSystem Specifications/Application Functions/SF009A Thermal Duty Cycle Protection)' '#SF009A_285' 'true' 'REQ: SF009A_285' '' } %GIDa_c154c904_67c1_4cef_84fc_7ec700beb4b5  OutDataTypeStr=int32
  DutyCycThermProtnFilt1Init : Fil/FilLpInit  RequirementInfo={'linktype_rmi_doors' '0000a52a (/E-STEER Core/SubSystem Specifications/Application Functions/SF009A Thermal Duty Cycle Protection)' '#SF009A_117' 'true' 'REQ: SF009A_117' '' } %GIDa_0e8bfc14_723b_4891_b23d_ae1d7fa99241  Ic=0  Ts=ARCHGLBPRM_100MILLISEC_SEC_F32  Freq=FIL1LPFILFRQ_HZ_F32  StVar=Fil1ValStVari
  DutyCycThermProtnFilt2Init : Fil/FilLpInit  RequirementInfo={'linktype_rmi_doors' '0000a52a (/E-STEER Core/SubSystem Specifications/Application Functions/SF009A Thermal Duty Cycle Protection)' '#SF009A_117' 'true' 'REQ: SF009A_117' '' } %GIDa_e86bde5d_0b0e_456d_9f54_4bce79809900  Ic=0  Ts=ARCHGLBPRM_100MILLISEC_SEC_F32  Freq=FIL2LPFILFRQ_HZ_F32  StVar=Fil2ValStVari
  DutyCycThermProtnFilt3Init : Fil/FilLpInit  RequirementInfo={'linktype_rmi_doors' '0000a52a (/E-STEER Core/SubSystem Specifications/Application Functions/SF009A Thermal Duty Cycle Protection)' '#SF009A_117' 'true' 'REQ: SF009A_117' '' } %GIDa_da5eaa20_ceb2_422b_a114_91fce26b7226  Ic=0  Ts=ARCHGLBPRM_100MILLISEC_SEC_F32  Freq=FIL3LPFILFRQ_HZ_F32  StVar=Fild3Val
  DutyCycThermProtnFilt4Init : Fil/FilLpInit  RequirementInfo={'linktype_rmi_doors' '0000a52a (/E-STEER Core/SubSystem Specifications/Application Functions/SF009A Thermal Duty Cycle Protection)' '#SF009A_117' 'true' 'REQ: SF009A_117' '' } %GIDa_1e09f253_99fc_475f_b7b1_2363ca9043b7  Ic=0  Ts=ARCHGLBPRM_100MILLISEC_SEC_F32  Freq=FIL4LPFILFRQ_HZ_F32  StVar=Fild4Val
  DutyCycThermProtnFilt5Init : Fil/FilLpInit  RequirementInfo={'linktype_rmi_doors' '0000a52a (/E-STEER Core/SubSystem Specifications/Application Functions/SF009A Thermal Duty Cycle Protection)' '#SF009A_117' 'true' 'REQ: SF009A_117' '' } %GIDa_04d09b42_a90f_4fcf_be3c_26f243fe1181  Ic=0  Ts=ARCHGLBPRM_100MILLISEC_SEC_F32  Freq=FIL5LPFILFRQ_HZ_F32  StVar=Fild5Val
  DutyCycThermProtnFilt6Init : Fil/FilLpInit  RequirementInfo={'linktype_rmi_doors' '0000a52a (/E-STEER Core/SubSystem Specifications/Application Functions/SF009A Thermal Duty Cycle Protection)' '#SF009A_117' 'true' 'REQ: SF009A_117' '' } %GIDa_17f03d4f_452d_42f6_8cbd_b04edf592325  Ic=0  Ts=ARCHGLBPRM_100MILLISEC_SEC_F32  Freq=FIL6LPFILFRQ_HZ_F32  StVar=Fild6Val
  Enumerated Constant : simulink/Sources/Enumerated Constant  RequirementInfo={'linktype_rmi_doors' '0000a52a (/E-STEER Core/SubSystem Specifications/Application Functions/SF009A Thermal Duty Cycle Protection)' '#SF009A_285' 'true' 'REQ: SF009A_285' '' } %GIDa_adac693a_e803_425c_a30d_199718a98f3c  OutDataTypeStr=Enum: NvmGetErrSts1  Value=NvmGetErrSts1.REQUEST_OK  SampleTime=inf
  FilStVal_SetRamBlockStatus : Subsystem
  Get Error Status : NxtrNvM/Get Error Status  RequirementInfo={'linktype_rmi_doors' '0000a52a (/E-STEER Core/SubSystem Specifications/Application Functions/SF009A Thermal Duty Cycle Protection)' '#SF009A_285' 'true' 'REQ: SF009A_285' '' } %GIDa_aa49604e_1ff8_4c6f_bfbb_5888efbf4cb8  FuncName=Get Error Status  NvMBlockName=FilStVal  VoidFuncRtn=on  ReqResPtr_DSN=NvMGES_ReqResPtr  Return_DSN=NvMGES_ReqResPtr1
      settings: AttributesFormatString=%<FuncName>
  If : If  RequirementInfo={'linktype_rmi_doors' '0000a52a (/E-STEER Core/SubSystem Specifications/Application Functions/SF009A Thermal Duty Cycle Protection)' '#SF009A_285' 'true' 'REQ: SF009A_285' '' } %GIDa_8c6cd8b0_ce48_4d5a_9d1b_7bcef7ec6fa2  Priority=1  IfExpression=u1
      settings: AttributesFormatString=Priority =%<Priority>
  NVM_NOK : Subsystem  RequirementInfo={'linktype_rmi_doors' '0000a52a (/E-STEER Core/SubSystem Specifications/Application Functions/SF009A Thermal Duty Cycle Protection)' '#SF009A_205' 'true' 'REQ: SF009A_205' '' } %GIDa_4f43ad0f_1af8_4a8c_a031_3900765618c8  TreatAsAtomicUnit=on
  NVM_Ok : Subsystem  RequirementInfo={'linktype_rmi_doors' '0000a52a (/E-STEER Core/SubSystem Specifications/Application Functions/SF009A Thermal Duty Cycle Protection)' '#SF009A_205' 'true' 'REQ: SF009A_205' '' } %GIDa_63a0e7b6_7be4_4cfe_a821_614fa63f81ac  TreatAsAtomicUnit=on
  PowerOnTasks : Subsystem  RequirementInfo={} %GIDa_e1b87dcc_ac2c_4e13_9d90_dc0935cdb67e
  Relational Operator4 : RelationalOperator  RequirementInfo={'linktype_rmi_doors' '0000a52a (/E-STEER Core/SubSystem Specifications/Application Functions/SF009A Thermal Duty Cycle Protection)' '#SF009A_285' 'true' 'REQ: SF009A_285' '' } %GIDa_c9b70987_85cc_4c3f_84c6_6174b6ee84db  Operator=~=  OutDataTypeStr=boolean
  SetInitialValueOfAbsTempLimitSlew : Subsystem  TreatAsAtomicUnit=on
  SetInitialValueOfLstTblValRateLimrStVari : Subsystem  TreatAsAtomicUnit=on
  FilStVariReInitFlg : Outport
  wires:
  Constant/1 -> Data Store Write/1
  Data Store Read/1 -> Data Store Write1/1
  Data Store Read1/1 -> Data Store Write2/1
  Data Store Read2/1 -> Data Store Write3/1
  Data Store Read3/1 -> Data Store Write4/1
  DutyCycThermProtnDi/1 -> PowerOnTasks/3(DutyCycThermProtnDi)
  VehTiVld/1 -> PowerOnTasks/2(VehTiVld)
  IgnTiOff/1 -> PowerOnTasks/1(IgnTiOff)
  PowerOnTasks/1(FilStVariReInitFlg) -> FilStVariReInitFlg/1
  Constant1/1 -> FilStVal_SetRamBlockStatus/1(BlockChanged)
  Constant2/1 -> Data Store Write5/1
  If/1 -> NVM_NOK/Action
  If/2 -> NVM_Ok/Action
  Get Error Status/1 -> Data Type Conversion1/1
  Enumerated Constant/1 -> Relational Operator4/2
  Data Type Conversion/1 -> Relational Operator4/1
  Data Type Conversion1/1 -> Data Type Conversion/1
  Relational Operator4/1 -> If/1

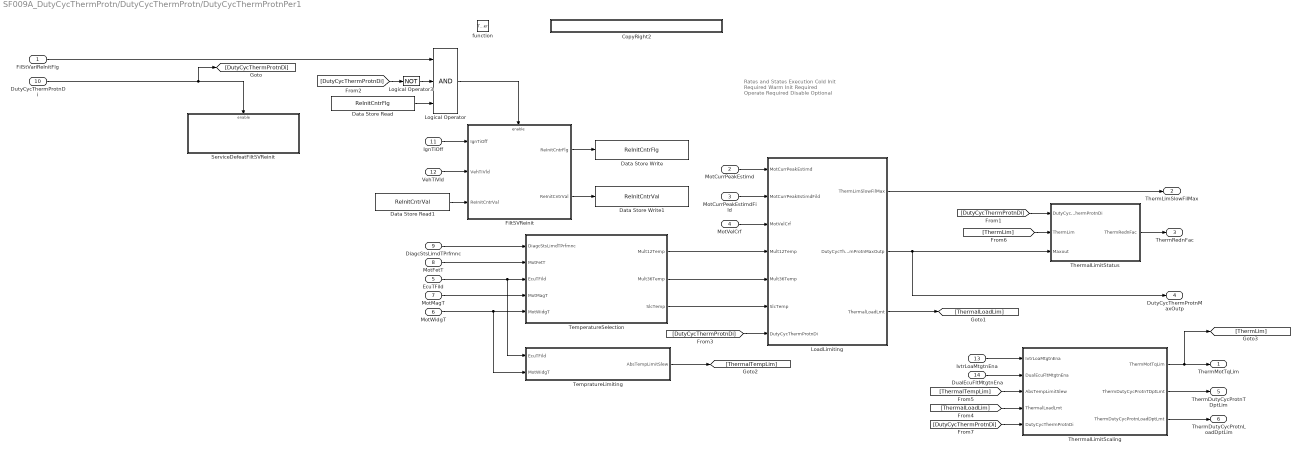
== system SF009A_DutyCycThermProtn/DutyCycThermProtn/DutyCycThermProtnPer1 ==
  note: Rates and States Execution
      |   Cold Init     Required
      |   Warm Init   Required
      |   Operate      Required
      |   Disable      Optional
  FilStVariReInitFlg : Inport
  MotCurrPeakEstimd : Inport  Port=2
  MotCurrPeakEstimdFild : Inport  Port=3
  MotVelCrf : Inport  Port=4
  EcuTFild : Inport  Port=5
  MotWidgT : Inport  Port=6
  MotMagT : Inport  Port=7
  MotFetT : Inport  Port=8
  DiagcStsLimdTPrfmnc : Inport  Port=9
  DutyCycThermProtnDi : Inport  Port=10
  IgnTiOff : Inport  Port=11
  VehTiVld : Inport  Port=12
  IvtrLoaMtgtnEna : Inport  Port=13
  DualEcuFltMtgtnEna : Inport  Port=14
  function : TriggerPort  TriggerType=function-call
  CopyRight2 : Subsystem  Description=|  mask(Copyright Information){none=on}
      | Copyright info block.                                               
      |                                                                     
      | Place copyright information at the top of every subsystem in design.
      mask prompts: none "No parameters"
      mask help: Place copyright information at the top of every subsystem in design.
      mask Display:
      | NxtrConf = 'Nexteer Confidential';
      | 
      | sys = bdroot; %handle for the current model ("system")
      | first = get_param(sys,'Created');
      | if(isempty(first))
      |     first = datestr(now,'yyyy');
      | else
      |     first = first(end-3:end);  %year is last four digits
      | end
      | 
      | last = get_param(sys,'LastModifiedDate');
      | if isempty(last)
      |     last = datestr(now,'yyyy');
      | else
      |     last = last(end-3:end);
      | end
      | 
      | if strcmp(first,last)
      |     fprintf('%s -- Copyright %s Nexteer',NxtrConf,first)
      | else
      |     fprintf('%s -- %s%s- %s Nexteer',NxtrConf,char(169),first,last)
      | end
  Data Store Read : DataStoreRead  DataStoreName=ReInitCntrFlg
  Data Store Read1 : DataStoreRead  DataStoreName=ReInitCntrVal
  Data Store Write : DataStoreWrite  DataStoreName=ReInitCntrFlg
  Data Store Write1 : DataStoreWrite  DataStoreName=ReInitCntrVal
  FiltSVReinit : Subsystem  RequirementInfo={'linktype_rmi_doors' '0000a52a (/E-STEER Core/SubSystem Specifications/Application Functions/SF009A Thermal Duty Cycle Protection)' '#SF009A_138' 'true' 'REQ: SF009A_138' '' } %GIDa_f037a2ca_95ef_4c06_a841_0ea43f8e71a8
  LoadLimiting : Subsystem
  Logical Operator : Logic  Inputs=3  AllPortsSameDT=off  OutDataTypeStr=boolean
  Logical Operator3 : Logic  Operator=NOT  Inputs=1  AllPortsSameDT=off  OutDataTypeStr=boolean
  ServiceDefeatFiltSVReinit : Subsystem  RequirementInfo={} %GIDa_c4f3c208_ab6c_44db_9d7b_87c98a9094da
  TemperatureSelection : Subsystem  RequirementInfo={} %GIDa_834c6c59_b5eb_40dc_b0a0_0f78997f326f
  TempratureLimiting : Subsystem  RequirementInfo={} %GIDa_e6f9c2a3_9cf9_4de2_87ea_c958f0e34b85
  ThermalLimitStatus : Subsystem
  TherrmalLimitScaling : Subsystem  RequirementInfo={} %GIDa_6c00c7b2_b56e_4406_a298_18898792b3b5
  ThermMotTqLim : Outport
  ThermLimSlowFilMax : Outport  Port=2
  ThermRednFac : Outport  Port=3
  DutyCycThermProtnMaxOutp : Outport  Port=4
  ThermDutyCycProtnTDptLim : Outport  Port=5
  ThermDutyCycProtnLoadDptLim : Outport  Port=6
  wires:
  TemperatureSelection/2(Mult36Temp) -> LoadLimiting/5(Mult36Temp)
  TemperatureSelection/1(Mult12Temp) -> LoadLimiting/4(Mult12Temp)
  TemperatureSelection/3(SlcTemp) -> LoadLimiting/6(SlcTemp)
  EcuTFild/1 -> TempratureLimiting/1(EcuTFild), TemperatureSelection/3(EcuTFild)
  MotWidgT/1 -> TempratureLimiting/2(MotWidgT), TemperatureSelection/5(MotWidgT)
  MotCurrPeakEstimd/1 -> LoadLimiting/1(MotCurrPeakEstimd)
  MotCurrPeakEstimdFild/1 -> LoadLimiting/2(MotCurrPeakEstimdFild)
  MotVelCrf/1 -> LoadLimiting/3(MotVelCrf)
  DiagcStsLimdTPrfmnc/1 -> TemperatureSelection/1(DiagcStsLimdTPrfmnc)
  MotFetT/1 -> TemperatureSelection/2(MotFetT)
  LoadLimiting/1(ThermLimSlowFilMax) -> ThermLimSlowFilMax/1
  MotMagT/1 -> TemperatureSelection/4(MotMagT)
  IgnTiOff/1 -> FiltSVReinit/1("IgnTiOff ")
  VehTiVld/1 -> FiltSVReinit/2(VehTiVld)
  Logical Operator/1 -> FiltSVReinit/Enable
  Logical Operator3/1 -> Logical Operator/2
  [DutyCycThermProtnDi] -> Logical Operator3/1
  DutyCycThermProtnDi/1 -> ServiceDefeatFiltSVReinit/Enable, [DutyCycThermProtnDi]
  FiltSVReinit/1(ReInitCntrFlg) -> Data Store Write/1
  Data Store Read/1 -> Logical Operator/3
  FiltSVReinit/2(ReInitCntrVal) -> Data Store Write1/1
  Data Store Read1/1 -> FiltSVReinit/3("ReInitCntrVal ")
  FilStVariReInitFlg/1 -> Logical Operator/1
  [DutyCycThermProtnDi] -> LoadLimiting/7(DutyCycThermProtnDi)
  LoadLimiting/3(ThermalLoadLmt) -> [ThermalLoadLim]
  TherrmalLimitScaling/1(ThermMotTqLim) -> [ThermLim], ThermMotTqLim/1
  LoadLimiting/2(DutyCycThermProtnMaxOutp) -> DutyCycThermProtnMaxOutp/1, ThermalLimitStatus/3(Maxout)
  TherrmalLimitScaling/2(ThermDutyCycProtnTDptLmt) -> ThermDutyCycProtnTDptLim/1
  TherrmalLimitScaling/3(ThermDutyCycProtnLoadDptLmt) -> ThermDutyCycProtnLoadDptLim/1
  [ThermalLoadLim] -> TherrmalLimitScaling/4(ThermalLoadLmt)
  TempratureLimiting/1(AbsTempLimitSlew) -> [ThermalTempLim]
  [ThermalTempLim] -> TherrmalLimitScaling/3(AbsTempLimitSlew)
  [ThermLim] -> ThermalLimitStatus/2(ThermLim)
  [DutyCycThermProtnDi] -> ThermalLimitStatus/1(DutyCycThermProtnDi)
  ThermalLimitStatus/1(ThermRednFac) -> ThermRednFac/1
  IvtrLoaMtgtnEna/1 -> TherrmalLimitScaling/1(IvtrLoaMtgtnEna)
  DualEcuFltMtgtnEna/1 -> TherrmalLimitScaling/2(DualEcuFltMtgtnEna)
  [DutyCycThermProtnDi] -> TherrmalLimitScaling/5(DutyCycThermProtnDi)

== system SF009A_DutyCycThermProtn/DutyCycThermProtn/DutyCycThermProtnInit1/CopyRight2 ==

== system SF009A_DutyCycThermProtn/DutyCycThermProtn/DutyCycThermProtnInit1/FilStVal_SetRamBlockStatus ==
  note: This is the block representing the client call
  BlockChanged : Inport
  CopyRight2 : Subsystem  Description=|  mask(Copyright Information){none=on}
      | Copyright info block.                                               
      |                                                                     
      | Place copyright information at the top of every subsystem in design.
      mask prompts: none "No parameters"
      mask help: Place copyright information at the top of every subsystem in design.
      mask Display:
      | NxtrConf = 'Nexteer Confidential';
      | 
      | sys = bdroot; %handle for the current model ("system")
      | first = get_param(sys,'Created');
      | if(isempty(first))
      |     first = datestr(now,'yyyy');
      | else
      |     first = first(end-3:end);  %year is last four digits
      | end
      | 
      | last = get_param(sys,'LastModifiedDate');
      | if isempty(last)
      |     last = datestr(now,'yyyy');
      | else
      |     last = last(end-3:end);
      | end
      | 
      | if strcmp(first,last)
      |     fprintf('%s -- Copyright %s Nexteer',NxtrConf,first)
      | else
      |     fprintf('%s -- %s%s- %s Nexteer',NxtrConf,char(169),first,last)
      | end
  Terminator : Terminator
  wires:
  BlockChanged/1 -> Terminator/1
